simulink model "LogicalOperator_TestGen5"  (R2017b)
settings: Solver=FixedStepDiscrete  StartTime=0.0  StopTime=10.0  RelTol=1e-3
settings Model: Creator=ktrinh  LastModifiedBy=ktrinh
settings DebuggingCC: ParameterOverflowMsg=none

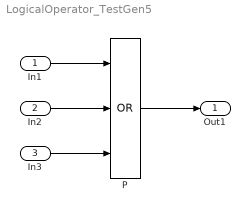
== system LogicalOperator_TestGen5 ==
  In1 : Inport  OutDataTypeStr=boolean  PortDimensions=1
  In2 : Inport  Port=2  OutDataTypeStr=boolean  PortDimensions=1
  In3 : Inport  Port=3  OutDataTypeStr=boolean  PortDimensions=1
  P : Logic  Operator=OR  Inputs=3  AllPortsSameDT=off  OutDataTypeStr=boolean
  Out1 : Outport
  wires:
  In1/1 -> P/1
  In2/1 -> P/2
  In3/1 -> P/3
  P/1 -> Out1/1
